simulink model "Part_1"  (R2017b)
settings: Solver=VariableStepAuto  StartTime=0.0  StopTime=0  RelTol=1e-3
libraries: dspsigops x1
settings Model: Creator=Alireza Rafiee  LastModifiedBy=Alireza Rafiee
settings DataIOCC: ReturnWorkspaceOutputs=on
settings SFSimCC: SimUseLocalCustomCode=on
settings RTWCC: RTWUseLocalCustomCode=on

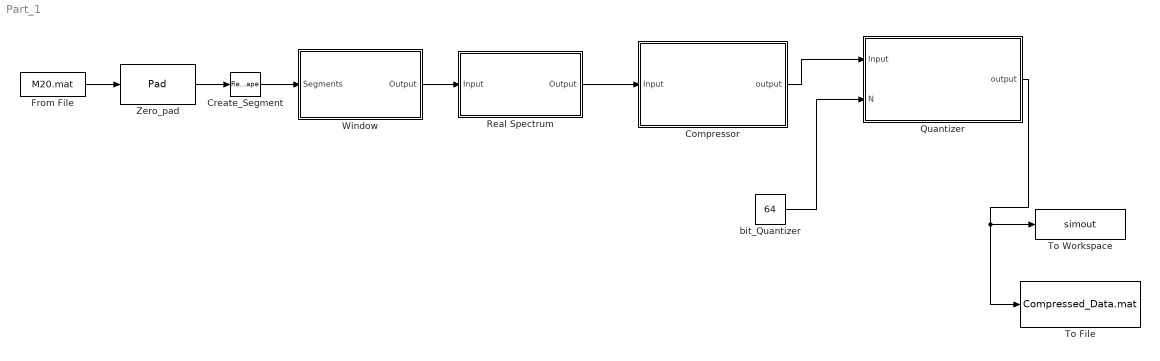
== system Part_1 ==
  Compressor : MATLAB Function  TreatAsAtomicUnit=on
  Create_Segment : Reshape  OutputDimensionality=Customize  OutputDimensions=[400,150]
  From File : FromFile  FileName=M20.mat  SampleTime=0
  Quantizer : MATLAB Function  TreatAsAtomicUnit=on
  Real Spectrum : MATLAB Function  TreatAsAtomicUnit=on
  To File : ToFile  Filename=Compressed_Data.mat  MatrixName=Compressed_Data  SaveFormat=Timeseries
  To Workspace : ToWorkspace  VariableName=simout  SampleTime=-1
      settings: Save2DSignal=2-D array (concatenate along first dimension)
  Window : MATLAB Function  TreatAsAtomicUnit=on
  Zero_pad : dspsigops/Pad  padAlong=Rows  dimsToPad=1  valSrc=Specify via dialog  padVal=0  spec=Output size  padNumOutRowsSpecMethod=User-specified  numOutRows=301  padNumOutColsSpecMethod=User-specified  numOutCols=60000  isVarDimsMode=off  padBeginning=0  padEnd=0  outSizeMode=User-specified  outSize=1  padSigAt=End  trunc_flag=None  roundingMode=Floor  overflowMode=off  truncOrWrapMode=Truncate  wrap_flag=None
      settings: SourceProductBaseCode=DS
  bit_Quantizer : Constant  Value=64
  wires:
  Zero_pad/1 -> Create_Segment/1
  From File/1 -> Zero_pad/1
  Create_Segment/1 -> Window/1(Segments)
  Window/1(Output) -> Real Spectrum/1(Input)
  Real Spectrum/1(Output) -> Compressor/1(Input)
  Compressor/1(output) -> Quantizer/1(Input)
  bit_Quantizer/1 -> Quantizer/2(N)
  Quantizer/1(output) -> To Workspace/1, To File/1

== matlab function Part_1/Real Spectrum ==
  data: Input input; Output output
function Output = R_Cepstrum(Input)
L=0;
H=0;
[H,L]=size(Input);
Output=zeros(H,L);
i=0;
for i=1:1:L
   Output(:,i)=rceps(Input(:,i)); %real Cepstrum of input
end

== matlab function Part_1/Window ==
  data: Segments input; Output output
function Output = Window(Segments)
L=0;
H=0;
[H,L]=size(Segments);
Output=zeros(H,L);
window=zeros(H,1);
window=hamming(H);%Hamming Window
i=0;
for i=1:1:L
   Output(:,i)=Segments(:,i).*window; %multiple window and Segments
end

== matlab function Part_1/Compressor ==
  data: Input input; output output
function output = Compressor(Input)
L=0;
H=0;
Save_len=15;
[H,L]=size(Input);
Output_pre=zeros((Save_len+2),L);
Output=zeros((Save_len+2),L);
Temp=zeros(H/2-Save_len,1);
pitch_amp=0;%pitch amplitude
pitch_loc=0;%pitch location
i=0;
for i=1:1:L
    for k=1:1:Save_len
   Output_pre(k,i)=Input(k,i);%save the begin of cepstrum
    end
    Temp=Input(Save_len+1:1:H/2,i);%pick the frist half of Cepstrum without the starting data
    [pitch_amp,pitch_loc]=max(abs(Temp));
    pitch_amp=Temp(pitch_loc);%determine pitch amplitude
    pitch_loc=pitch_loc+Save_len;%determine pitch location
    Output_pre(Save_len+1,i)=pitch_loc;%Save pitch
    Output_pre(Save_len+2,i)=pitch_amp;
end
output = Output_pre;

== matlab function Part_1/Quantizer ==
  data: Input input; output output; N input
function output = Quantizer(Input,N)
L=0;
H=0;
[H,L]=size(Input);
Output_pre=zeros(H,L);
Output=zeros(H,L);
i=0;
X_max=0;
Delta=0;
X_max=max(max(abs(Input)));
Delta=2*X_max/(2^N);
for i=1:1:L
    Output_pre(:,i)=Delta*round(Input(:,i)/Delta);%Quantizer
end
output = Output_pre;
